simulink model "Subsystems_Tests"  (R2023b)
settings: Solver=VariableStepAuto  StartTime=0.0  StopTime=10  RelTol=1e-3
values from neighbouring files (symbols this model uses):
  a = 1.35    [Parameters.m]
  b = 1.5    [Parameters.m]
  Csc = 600    [Parameters.m]
  Cse = 1200    [Parameters.m]
  g = 9.81    [Parameters.m]
  I = 650    [Parameters.m]
  Kt = 14e4    (= 140000)    [Parameters.m]
  Mb = 700    [Parameters.m]
  Mw = 20    [Parameters.m]
libraries: CarModelLibrary x12
settings Model: Creator=fb552  LastModifiedBy=franc
settings SolverCC: AlgebraicLoopSolver=TrustRegion
settings DebuggingCC: UnconnectedInputMsg=warning  UnconnectedOutputMsg=warning  UnconnectedLineMsg=warning
settings ModelReferenceCC: EnableRefExpFcnMdlSchedulingChecks=on

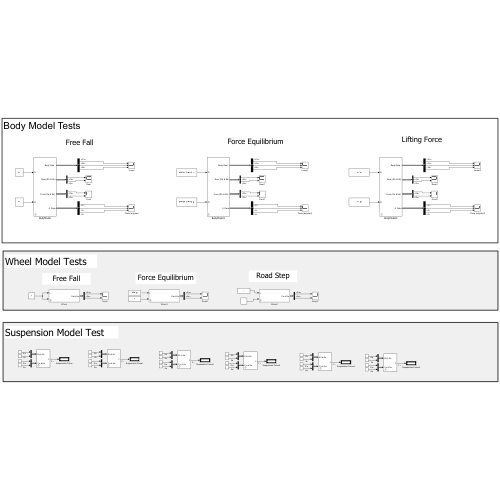
[thumbnail: Simulink's stored preview of the top-level diagram]
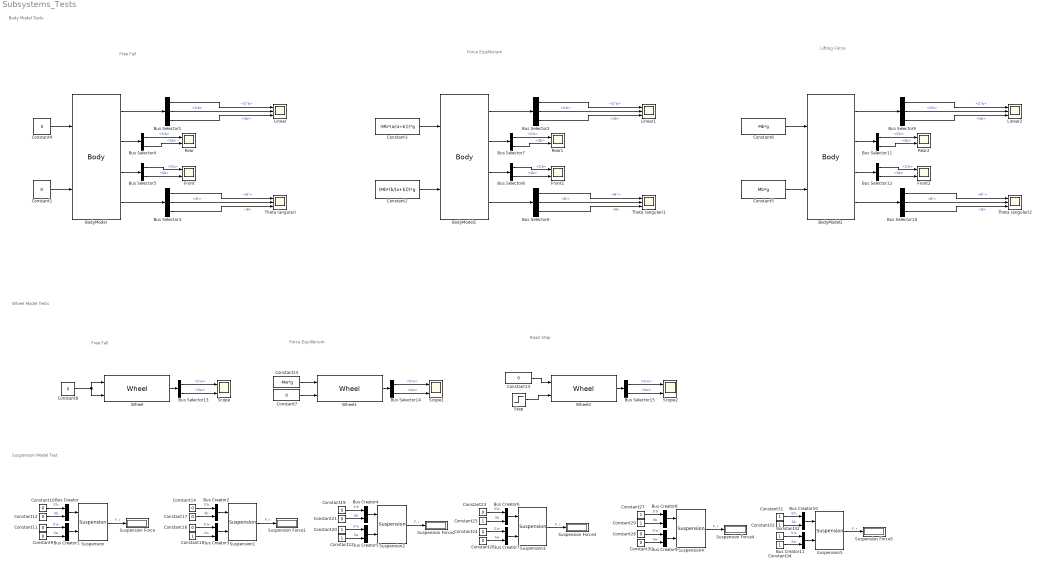
== system Subsystems_Tests ==
  note: Body Model Tests
  note: Force Equilibrium
  note: Free Fall
  note: Lifting Force
  note: Wheel Model Tests
  note: Suspension Model Test
  note: Free Fall
  note: Force Equilibrium
  note: Road Step
  BodyModel : CarModelLibrary/Body  mb=Mb  I=I  a=a  b=b
  BodyModel1 : CarModelLibrary/Body  mb=Mb  I=I  a=a  b=b
  BodyModel2 : CarModelLibrary/Body  mb=Mb  I=I  a=a  b=b
  Bus Creator{,1..11} (12 alike) : BusCreator  Inputs=2
  Bus Selector1 : BusSelector  OutputSignals=S''b,S'b,Sb
  Bus Selector10 : BusSelector  OutputSignals=θ'',θ',θ
  Bus Selector{4..5,7..8,11..12} (6 alike) : BusSelector  OutputSignals=S'b,Sb
  Bus Selector13 : BusSelector  OutputSignals=S'w,Sw
  Bus Selector14 : BusSelector  OutputSignals=S'w,Sw
  Bus Selector15 : BusSelector  OutputSignals=S'w,Sw
  Bus Selector2 : BusSelector  OutputSignals=S''b,S'b,Sb
  Bus Selector3 : BusSelector  OutputSignals=θ'',θ',θ
  Bus Selector6 : BusSelector  OutputSignals=θ'',θ',θ
  Bus Selector9 : BusSelector  OutputSignals=S''b,S'b,Sb
  Constant{1,4,7..14,16..17,19,21,23..24,26,28,30} (19 alike) : Constant  Value=0
  Constant15 : Constant  Value=-Mw*g
  Constant{18,20,22,25,27,29,31..34} (10 alike) : Constant
  Constant2 : Constant  Value=(Mb*(b/(a+b)))*g
  Constant3 : Constant  Value=(Mb*(a/(a+b)))*g
  Constant5 : Constant  Value=Mb*g
  Constant6 : Constant  Value=Mb*g
  Front : Scope  NumInputPorts=2
  Front1 : Scope  NumInputPorts=2
  Front2 : Scope  NumInputPorts=2
  Linear : Scope  NumInputPorts=3
  Linear1 : Scope  NumInputPorts=3
  Linear2 : Scope  NumInputPorts=3
  Rear : Scope  NumInputPorts=2
  Rear1 : Scope  NumInputPorts=2
  Rear2 : Scope  NumInputPorts=2
  Scope : Scope  NumInputPorts=2
  Scope1 : Scope  NumInputPorts=2
  Scope2 : Scope  NumInputPorts=2
  Step : Step  SampleTime=0
  Suspension{,1..5} (6 alike) : CarModelLibrary/Suspension  ks=Ks  ksstiff=1  x0=x0  csb=(Csc+Cse)/2  csr=(Csc+Cse)/2
  Suspension Force{,1..5} (6 alike) : Display
  Theta (angular) : Scope  NumInputPorts=3
  Theta (angular)1 : Scope  NumInputPorts=3
  Theta (angular)2 : Scope  NumInputPorts=3
  Wheel : CarModelLibrary/Wheel  mw=Mw  Kt=0  g=g
      link override Constant: Value=mw*g
  Wheel1 : CarModelLibrary/Wheel  mw=Mw  Kt=0  g=g
      link override Constant: Value=mw*g
  Wheel2 : CarModelLibrary/Wheel  mw=Mw  Kt=Kt  g=0
  wires:
  Constant4/1 -> BodyModel/1
  Constant1/1 -> BodyModel/2
  BodyModel/4 -> Bus Selector3/1
  BodyModel/1 -> Bus Selector1/1
  Bus Selector1/3 -> Linear/3  "<Sb>"
  Bus Selector1/1 -> Linear/1  "<S''b>"
  Bus Selector1/2 -> Linear/2  "<S'b>"
  Bus Selector3/2 -> Theta (angular)/2  "<θ'>"
  BodyModel/3 -> Bus Selector5/1
  BodyModel/2 -> Bus Selector4/1
  Bus Selector4/1 -> Rear/1  "<S'b>"
  Bus Selector4/2 -> Rear/2  "<Sb>"
  Bus Selector5/2 -> Front/2  "<Sb>"
  Bus Selector5/1 -> Front/1  "<S'b>"
  Bus Selector7/1 -> Rear1/1  "<S'b>"
  Bus Selector6/2 -> Theta (angular)1/2  "<θ'>"
  Bus Selector2/3 -> Linear1/3  "<Sb>"
  Bus Selector8/1 -> Front1/1  "<S'b>"
  BodyModel1/3 -> Bus Selector8/1
  BodyModel1/2 -> Bus Selector7/1
  BodyModel1/4 -> Bus Selector6/1
  Bus Selector2/1 -> Linear1/1  "<S''b>"
  Bus Selector2/2 -> Linear1/2  "<S'b>"
  Bus Selector8/2 -> Front1/2  "<Sb>"
  Constant2/1 -> BodyModel1/2
  Bus Selector7/2 -> Rear1/2  "<Sb>"
  Constant3/1 -> BodyModel1/1
  BodyModel1/1 -> Bus Selector2/1
  Bus Selector3/1 -> Theta (angular)/1  "<θ''>"
  Bus Selector3/3 -> Theta (angular)/3  "<θ>"
  Bus Selector6/3 -> Theta (angular)1/3  "<θ>"
  Bus Selector6/1 -> Theta (angular)1/1  "<θ''>"
  Constant6/1 -> BodyModel2/1
  Bus Selector9/3 -> Linear2/3  "<Sb>"
  Bus Selector10/2 -> Theta (angular)2/2  "<θ'>"
  Bus Selector11/1 -> Rear2/1  "<S'b>"
  Constant5/1 -> BodyModel2/2
  Bus Selector12/2 -> Front2/2  "<Sb>"
  Bus Selector11/2 -> Rear2/2  "<Sb>"
  BodyModel2/4 -> Bus Selector10/1
  BodyModel2/1 -> Bus Selector9/1
  BodyModel2/2 -> Bus Selector11/1
  BodyModel2/3 -> Bus Selector12/1
  Bus Selector9/1 -> Linear2/1  "<S''b>"
  Bus Selector12/1 -> Front2/1  "<S'b>"
  Bus Selector9/2 -> Linear2/2  "<S'b>"
  Bus Selector10/1 -> Theta (angular)2/1  "<θ''>"
  Bus Selector10/3 -> Theta (angular)2/3  "<θ>"
  Constant8/1 -> Wheel/2, Wheel/1
  Suspension/1 -> Suspension Force/1  "F, r"
  Constant10/1 -> Bus Creator/1  "S'b"
  Constant11/1 -> Bus Creator1/1  "S'w"
  Bus Creator1/1 -> Suspension/2
  Bus Creator/1 -> Suspension/1
  Wheel/1 -> Bus Selector13/1
  Bus Selector13/1 -> Scope/1  "<S'w>"
  Bus Selector13/2 -> Scope/2  "<Sw>"
  Wheel1/1 -> Bus Selector14/1
  Constant15/1 -> Wheel1/1
  Bus Selector14/1 -> Scope1/1  "<S'w>"
  Bus Selector14/2 -> Scope1/2  "<Sw>"
  Constant7/1 -> Wheel1/2
  Bus Selector15/1 -> Scope2/1  "<S'w>"
  Bus Selector15/2 -> Scope2/2  "<Sw>"
  Constant13/1 -> Wheel2/1
  Wheel2/1 -> Bus Selector15/1
  Step/1 -> Wheel2/2
  Constant9/1 -> Bus Creator1/2  "Sw"
  Constant12/1 -> Bus Creator/2  "Sb"
  Constant14/1 -> Bus Creator2/1  "S'b"
  Bus Creator3/1 -> Suspension1/2
  Suspension1/1 -> Suspension Force1/1  "F, r"
  Constant18/1 -> Bus Creator3/2  "Sw"
  Bus Creator2/1 -> Suspension1/1
  Constant17/1 -> Bus Creator2/2  "Sb"
  Constant16/1 -> Bus Creator3/1  "S'w"
  Constant19/1 -> Bus Creator4/1  "S'b"
  Bus Creator5/1 -> Suspension2/2
  Suspension2/1 -> Suspension Force2/1  "F, r"
  Constant22/1 -> Bus Creator5/2  "Sw"
  Bus Creator4/1 -> Suspension2/1
  Constant21/1 -> Bus Creator4/2  "Sb"
  Constant20/1 -> Bus Creator5/1  "S'w"
  Constant23/1 -> Bus Creator6/1  "S'b"
  Bus Creator7/1 -> Suspension3/2
  Suspension3/1 -> Suspension Force3/1  "F, r"
  Constant26/1 -> Bus Creator7/2  "Sw"
  Bus Creator6/1 -> Suspension3/1
  Constant25/1 -> Bus Creator6/2  "Sb"
  Constant24/1 -> Bus Creator7/1  "S'w"
  Constant27/1 -> Bus Creator8/1  "S'b"
  Bus Creator9/1 -> Suspension4/2
  Suspension4/1 -> Suspension Force4/1  "F, r"
  Constant30/1 -> Bus Creator9/2  "Sw"
  Bus Creator8/1 -> Suspension4/1
  Constant29/1 -> Bus Creator8/2  "Sb"
  Constant28/1 -> Bus Creator9/1  "S'w"
  Constant31/1 -> Bus Creator10/1  "S'b"
  Bus Creator11/1 -> Suspension5/2
  Suspension5/1 -> Suspension Force5/1  "F, r"
  Constant34/1 -> Bus Creator11/2  "Sw"
  Bus Creator10/1 -> Suspension5/1
  Constant33/1 -> Bus Creator10/2  "Sb"
  Constant32/1 -> Bus Creator11/1  "S'w"
